simulink model "gru_FL"  (R2020a)
settings: Solver=FixedStepAuto  StartTime=0.0  StopTime=Inf  FixedStep=0.001  MaxStep=0.01  RelTol=1e-3
InitFcn:
  | init_gru
StopFcn:
  | %stop_gru
values from neighbouring files (symbols this model uses):
  centro = [points(1); points(2)]    [init_gru.m]
  K1 = [20; 20]    [init_gru.m]
  K2 = [100; 100]    [init_gru.m]
  K3 = [10; 10]    [init_gru.m]
  L_dot_iniziale = 0    [init_gru.m]
  L_iniziale = 2    [init_gru.m]
  Lsofar = [Lsofar; sum(Lenghts)]    [init_gru.m]
  Ltot = sum(Lenghts)    [init_gru.m]
  n_p = length(points)    [init_gru.m]
  phi_dot_iniziale = 360/180*pi    (= 6.28318530718)    [init_gru.m]
  phi_iniziale = 30/180*pi    (= 0.523598775598)    [init_gru.m]
  theta_dot_iniziale = pi/8    (= 0.392699081699)    [init_gru.m]
  theta_iniziale = 20/180*pi    (= 0.349065850399)    [init_gru.m]
  theta_rette = [theta_rette ; theta_rette(n_p-2)+pi]    [init_gru.m]
  v_r = v_rif    (= 1)    [init_gru.m]
  x_M_finale = points(1)    [init_gru.m]
  x_M_iniziale = x_M_iniziale + offset_iniziale    [init_gru.m]
  x_t_dot_iniziale = 0    [init_gru.m]
  x_t_iniziale = 0    [init_gru.m]
  xp = points(:,1)    [init_gru.m]
  y_M_finale = points(2)    [init_gru.m]
  y_M_iniziale = y_M_iniziale + offset_iniziale*2    [init_gru.m]
  y_t_dot_iniziale = 0    [init_gru.m]
  y_t_iniziale = 0    [init_gru.m]
  yp = points(:,2)    [init_gru.m]
undefined symbols (not defined in the file or in its folder): indexclot, Lsofarclot
libraries: simulink x1
settings Model: Creator=Andrea_Ferroni  LastModifiedBy=Francesco

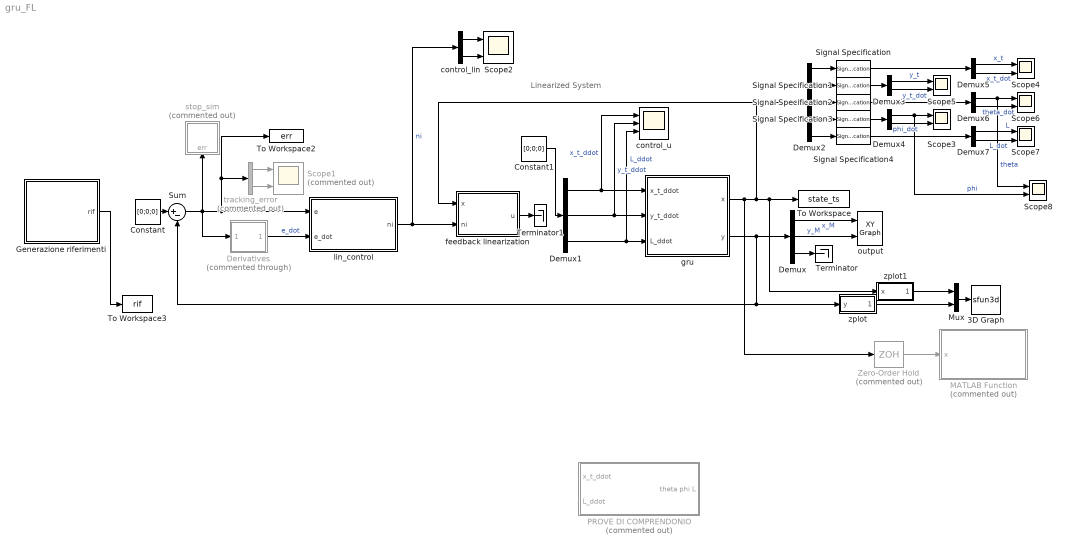
== system gru_FL ==
  note: Linearized System
  3D Graph : S-Function  LoadFcn=if exist('sfun3d','file'), sfun3d([],[],[],'LoadBlock'); end  FunctionName=sfun3d  Parameters=ax,T,np,cp,gd,ls,mk,mx,hd,tb  SFunctionDeploymentMode=off  EnableBusSupport=off  mask(3D Graph){np=2, ax=[-3 3 -3 3 -3 0.5], mx=1e4, T=0.1, cp=[3 2 1], gd=on, hd=off, tb=off, ls=-, mk=none}
      mask prompts: np "Number of moving points (lines)"; ax "Range: [xmin xmax  ymin ymax zmin zmax]"; mx "Max number of points in each line"; T "Sampling Time"; cp "Camera position (use [0 0 1] for 2D XY view)"; gd "Grid (on|off)"; hd "HeadMarkers (on|off)"; tb "Toolbar (on|off)"; ls "LineStyle"; mk "LineMarker"
      mask help:
      | This block plots the position of several points in the XYZ space. The input contains the coordinates of all the points (x1,y1,z1,x2,y2,z2,...).
      | The number of moving points (lines), the XYZ ranges, sampling time, camera position, and grid (among other things) can be set as mask parameters.
      settings: CopyFcn=if exist('sfun3d','file'), sfun3d([],[],[],'CopyBlock'); end  DeleteFcn=if exist('sfun3d','file'), sfun3d([],[],[],'DeleteBlock'); end  NameChangeFcn=if exist('sfun3d','file'), sfun3d([],[],[],'NameChange'); end
      mask Help:
      | This block plots the position of several points in the XYZ space. The input contains the coordinates of all the points (x1,y1,z1,x2,y2,z2,...).
      | The number of moving points (lines), the XYZ ranges, sampling time, camera position, and grid (among other things) can be set as mask parameters.
      mask TypeOptions ls: - | -- | : | -. | none
      mask TypeOptions mk: none | . | + | o | * | x | square | diamond | v | ^ | > | < | pentagram | hexagram
      mask Display: plot([.05 .95 .95 .05 .05],[.45 .45 .95 .95 .45], 0.5+cos(0:0.1:2*pi)*0.3,0.7+sin(0:0.1:2*pi)*0.2)
  Constant : Constant  Value=[0;0;0]
  Constant1 : Constant  Value=[0;0;0]
  Demux : Demux  Outputs=3
  Demux1 : Demux  Outputs=3
  Demux2 : Demux  Outputs=5
  Demux{3..7} (5 alike) : Demux  Outputs=2
  Derivatives : Subsystem  Commented=through
  Generazione riferimenti : Subsystem  Variant=on
  MATLAB Function : MATLAB Function  Commented=on  TreatAsAtomicUnit=on
  Mux : Mux  Inputs=2
  PROVE DI COMPRENDONIO : Subsystem  Commented=on
  Scope1 : Scope  Commented=on  NumInputPorts=2
  Scope{2..8} (7 alike) : Scope  NumInputPorts=2
  Signal Specification{,1..4} (5 alike) : SignalSpecification  Dimensions=[2,1]
  Sum : Sum  Inputs=|+-
  Terminator : Terminator
  Terminator1 : Terminator
  To Workspace : ToWorkspace  VariableName=state_ts  SaveFormat=Timeseries  SampleTime=-1
  To Workspace2 : ToWorkspace  VariableName=err  SaveFormat=Timeseries  SampleTime=-1
  To Workspace3 : ToWorkspace  VariableName=rif  SaveFormat=Timeseries  SampleTime=-1
  Zero-Order Hold : ZeroOrderHold  Commented=on  SampleTime=1/10
  control_lin : Demux  Outputs=2
  control_u : Scope  NumInputPorts=3
  feedback linearization : MATLAB Function  TreatAsAtomicUnit=on
  gru : Subsystem
  lin_control : MATLAB Function  TreatAsAtomicUnit=on
  output : simulink/Sinks/XY Graph  xmin=-50  xmax=50  ymin=-50  ymax=50  st=-1
  stop_sim : Subsystem  Commented=on
  tracking_error : Demux  Commented=on  Outputs=2
  zplot : MATLAB Function  TreatAsAtomicUnit=on
  zplot1 : MATLAB Function  TreatAsAtomicUnit=on
  wires:
  gru/2(y) -> Sum/2, zplot/1(y), Demux/1
  lin_control/1(ni) -> control_lin/1, feedback linearization/2(ni)  "ni"
  Sum/1 -> Derivatives/1(In1), lin_control/1(e), tracking_error/1, To Workspace2/1, stop_sim/1(err)
  Derivatives/1(Out1) -> lin_control/2(e_dot)  "e_dot"
  Demux/1 -> output/1  "x_M"
  Demux/2 -> output/2  "y_M"
  tracking_error/1 -> Scope1/1
  tracking_error/2 -> Scope1/2
  Demux1/1 -> control_u/1, gru/1(x_t_ddot)  "x_t_ddot"
  Demux1/2 -> gru/2(y_t_ddot), control_u/2  "y_t_ddot"
  control_lin/2 -> Scope2/2
  control_lin/1 -> Scope2/1
  Generazione riferimenti/1(rif) -> To Workspace3/1
  Demux1/3 -> control_u/3, gru/3(L_ddot)  "L_ddot"
  Demux/3 -> Terminator/1
  Demux2/1 -> Signal Specification/1
  Demux2/2 -> Signal Specification1/1
  Signal Specification1/1 -> Demux3/1
  Demux2/3 -> Signal Specification2/1
  Demux2/4 -> Signal Specification3/1
  Demux2/5 -> Signal Specification4/1
  Demux3/1 -> Scope5/1  "y_t"
  Demux3/2 -> Scope5/2  "y_t_dot"
  Demux4/1 -> Scope8/2, Scope3/1  "phi"
  Demux4/2 -> Scope3/2  "phi_dot"
  Signal Specification3/1 -> Demux4/1
  Demux5/1 -> Scope4/1  "x_t"
  Demux5/2 -> Scope4/2  "x_t_dot"
  Signal Specification/1 -> Demux5/1
  Demux6/1 -> Scope8/1, Scope6/1  "theta"
  Demux6/2 -> Scope6/2  "theta_dot"
  Signal Specification2/1 -> Demux6/1
  Demux7/1 -> Scope7/1  "L"
  Demux7/2 -> Scope7/2  "L_dot"
  Signal Specification4/1 -> Demux7/1
  Constant/1 -> Sum/1
  Constant1/1 -> Demux1/1
  zplot/1(y_new) -> Mux/2
  Mux/1 -> 3D Graph/1
  zplot1/1(trailer_graph) -> Mux/1
  gru/1(x) -> Zero-Order Hold/1, feedback linearization/1(x), Demux2/1, zplot1/1(x), To Workspace/1
  Zero-Order Hold/1 -> MATLAB Function/1(x)
  feedback linearization/1(u) -> Terminator1/1

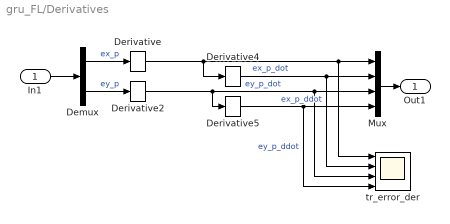
== system gru_FL/Derivatives ==
  In1 : Inport
  Demux : Demux  Outputs=2
  Derivative{,2,4..5} (4 alike) : Derivative  CoefficientInTFapproximation=1e10
  Mux : Mux
  tr_error_der : Scope  NumInputPorts=4
  Out1 : Outport
  wires:
  In1/1 -> Demux/1
  Demux/1 -> Derivative/1  "ex_p"
  Derivative/1 -> Derivative4/1, tr_error_der/1, Mux/1  "ex_p_dot"
  Demux/2 -> Derivative2/1  "ey_p"
  Mux/1 -> Out1/1
  Derivative4/1 -> tr_error_der/2, Mux/2  "ex_p_ddot"
  Derivative2/1 -> Derivative5/1, tr_error_der/3, Mux/3  "ey_p_dot"
  Derivative5/1 -> tr_error_der/4, Mux/4  "ey_p_ddot"

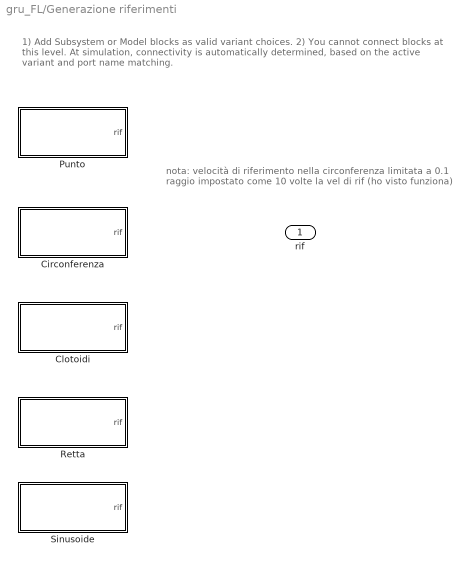
== system gru_FL/Generazione riferimenti ==
  note: nota:
      | velocità di riferimento nella circonferenza limitata a 0.1
      | raggio impostato come 10 volte la vel di rif (ho visto funziona)
  note: 1) Add Subsystem or Model blocks as valid variant choices.
      | 2) You cannot connect blocks at this level. At simulation, connectivity is automatically
      | determined, based on the active variant and port name matching.
  Circonferenza : Subsystem  VariantControl=Circonferenza
  Clotoidi : Subsystem  VariantControl=Clotoidi
  Punto : Subsystem  VariantControl=Punto
  Retta : Subsystem  VariantControl=Retta
  Sinusoide : Subsystem  VariantControl=Sinusoide
  rif : Outport

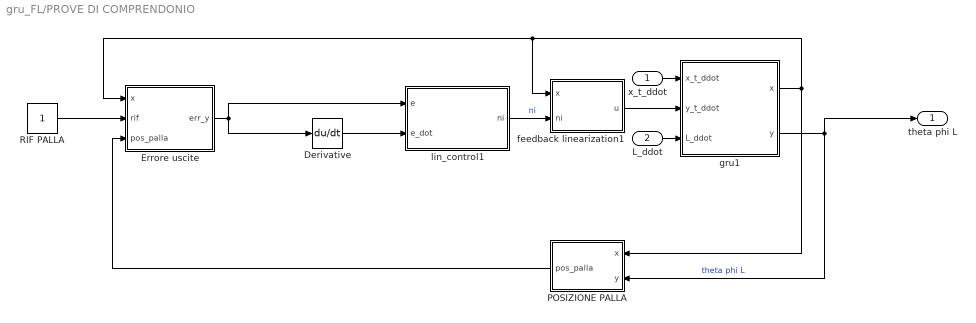
== system gru_FL/PROVE DI COMPRENDONIO ==
  x_t_ddot : Inport
  L_ddot : Inport  Port=2
  Derivative : Derivative
  Errore uscite : MATLAB Function  TreatAsAtomicUnit=on
  POSIZIONE PALLA : MATLAB Function  TreatAsAtomicUnit=on
  RIF PALLA : Constant
  feedback linearization1 : MATLAB Function  TreatAsAtomicUnit=on
  gru1 : Subsystem
  lin_control1 : MATLAB Function  TreatAsAtomicUnit=on
  theta phi L : Outport
  wires:
  Derivative/1 -> lin_control1/2(e_dot)
  lin_control1/1(ni) -> feedback linearization1/2(ni)  "ni"
  gru1/2(y) -> theta phi L/1, POSIZIONE PALLA/2(y)  "theta phi L"
  x_t_ddot/1 -> gru1/1(x_t_ddot)
  Errore uscite/1(err_y) -> lin_control1/1(e), Derivative/1
  POSIZIONE PALLA/1(pos_palla) -> Errore uscite/3(pos_palla)
  RIF PALLA/1 -> Errore uscite/2(rif)
  gru1/1(x) -> POSIZIONE PALLA/1(x), Errore uscite/1(x), feedback linearization1/1(x)
  feedback linearization1/1(u) -> gru1/2(y_t_ddot)
  L_ddot/1 -> gru1/3(L_ddot)

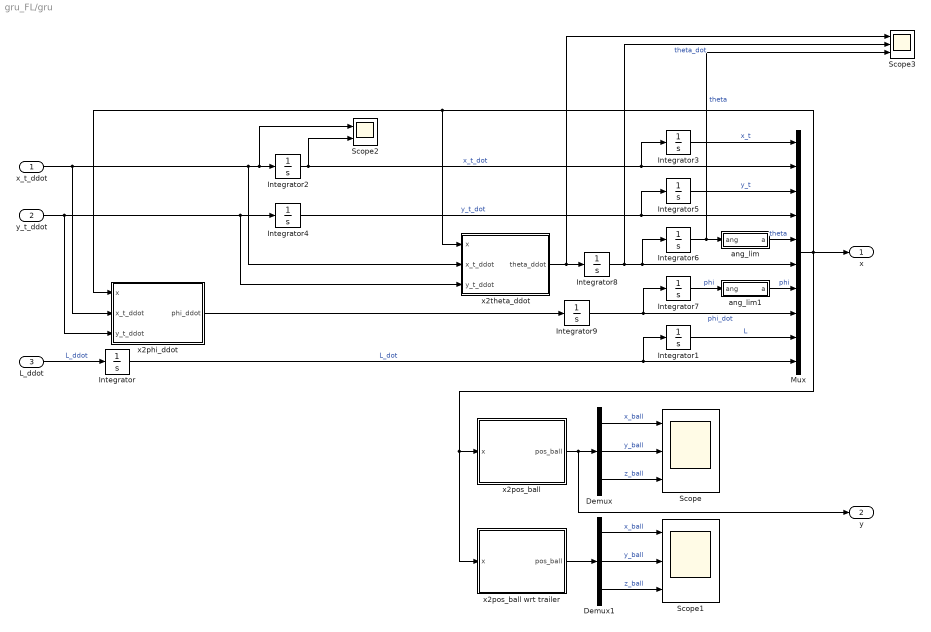
== system gru_FL/gru ==
  x_t_ddot : Inport
  y_t_ddot : Inport  Port=2
  L_ddot : Inport  Port=3
  Demux : Demux  Outputs=3
  Demux1 : Demux  Outputs=3
  Integrator : Integrator  InitialCondition=L_dot_iniziale
  Integrator1 : Integrator  InitialCondition=L_iniziale
  Integrator2 : Integrator  InitialCondition=x_t_dot_iniziale  UpperSaturationLimit=1e3  LowerSaturationLimit=-1e3
  Integrator3 : Integrator  InitialCondition=x_t_iniziale
  Integrator4 : Integrator  InitialCondition=y_t_dot_iniziale
  Integrator5 : Integrator  InitialCondition=y_t_iniziale
  Integrator6 : Integrator  InitialCondition=theta_iniziale
  Integrator7 : Integrator  InitialCondition=phi_iniziale
  Integrator8 : Integrator  InitialCondition=theta_dot_iniziale
  Integrator9 : Integrator  InitialCondition=phi_dot_iniziale
  Mux : Mux  Inputs=10
  Scope : Scope  NumInputPorts=3
  Scope1 : Scope  NumInputPorts=3
  Scope2 : Scope  NumInputPorts=2
  Scope3 : Scope  NumInputPorts=3
  ang_lim : MATLAB Function  TreatAsAtomicUnit=on
  ang_lim1 : MATLAB Function  TreatAsAtomicUnit=on
  x2phi_ddot : MATLAB Function  TreatAsAtomicUnit=on
  x2pos_ball : MATLAB Function  TreatAsAtomicUnit=on
  x2pos_ball wrt trailer : MATLAB Function  TreatAsAtomicUnit=on
  x2theta_ddot : MATLAB Function  TreatAsAtomicUnit=on
  x : Outport
  y : Outport  Port=2
  wires:
  x2pos_ball/1(pos_ball) -> y/1, Demux/1
  Integrator3/1 -> Mux/1  "x_t"
  Integrator2/1 -> Scope2/2, Integrator3/1, Mux/2  "x_t_dot"
  Integrator5/1 -> Mux/3  "y_t"
  Integrator4/1 -> Integrator5/1, Mux/4  "y_t_dot"
  Integrator6/1 -> Scope3/3, ang_lim/1(ang)  "theta"
  Integrator8/1 -> Scope3/2, Integrator6/1, Mux/6  "theta_dot"
  Integrator7/1 -> ang_lim1/1(ang)  "phi"
  Integrator9/1 -> Integrator7/1, Mux/8  "phi_dot"
  Integrator1/1 -> Mux/9  "L"
  L_ddot/1 -> Integrator/1  "L_ddot"
  Demux/1 -> Scope/1  "x_ball"
  Demux/2 -> Scope/2  "y_ball"
  Demux/3 -> Scope/3  "z_ball"
  Integrator/1 -> Integrator1/1, Mux/10  "L_dot"
  x_t_ddot/1 -> x2theta_ddot/2(x_t_ddot), Scope2/1, Integrator2/1, x2phi_ddot/2(x_t_ddot)
  y_t_ddot/1 -> x2theta_ddot/3(y_t_ddot), Integrator4/1, x2phi_ddot/3(y_t_ddot)
  x2theta_ddot/1(theta_ddot) -> Scope3/1, Integrator8/1
  x2phi_ddot/1(phi_ddot) -> Integrator9/1
  Mux/1 -> x2pos_ball wrt trailer/1(x), x2pos_ball/1(x), x2phi_ddot/1(x), x2theta_ddot/1(x), x/1
  Demux1/3 -> Scope1/3  "z_ball"
  Demux1/2 -> Scope1/2  "y_ball"
  Demux1/1 -> Scope1/1  "x_ball"
  x2pos_ball wrt trailer/1(pos_ball) -> Demux1/1
  ang_lim/1(a) -> Mux/5  "theta"
  ang_lim1/1(a) -> Mux/7  "phi"

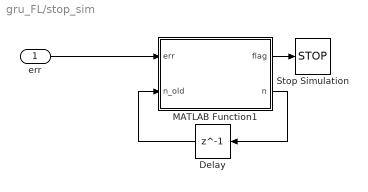
== system gru_FL/stop_sim ==
  err : Inport
  Delay : Delay  DelayLength=1
  MATLAB Function1 : MATLAB Function  TreatAsAtomicUnit=on
  Stop Simulation : Stop
  wires:
  MATLAB Function1/2(n) -> Delay/1
  MATLAB Function1/1(flag) -> Stop Simulation/1
  err/1 -> MATLAB Function1/1(err)
  Delay/1 -> MATLAB Function1/2(n_old)

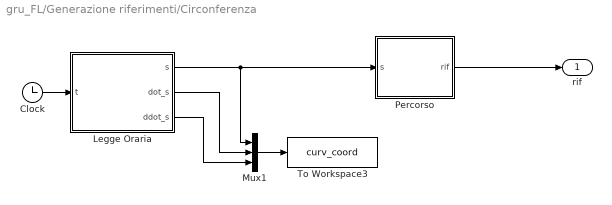
== system gru_FL/Generazione riferimenti/Circonferenza ==
  Clock : Clock
  Legge Oraria : MATLAB Function  TreatAsAtomicUnit=on
  Mux1 : Mux  Inputs=3
  Percorso : MATLAB Function  TreatAsAtomicUnit=on
  To Workspace3 : ToWorkspace  VariableName=curv_coord  SaveFormat=Timeseries  SampleTime=-1
  rif : Outport
  wires:
  Legge Oraria/2(dot_s) -> Mux1/2
  Clock/1 -> Legge Oraria/1(t)
  Mux1/1 -> To Workspace3/1
  Legge Oraria/3(ddot_s) -> Mux1/3
  Legge Oraria/1(s) -> Percorso/1(s), Mux1/1
  Percorso/1(rif) -> rif/1

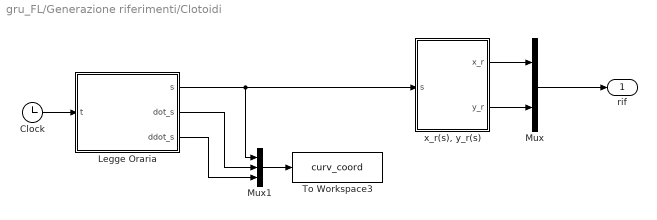
== system gru_FL/Generazione riferimenti/Clotoidi ==
  Clock : Clock
  Legge Oraria : MATLAB Function  TreatAsAtomicUnit=on
  Mux : Mux  Inputs=2
  Mux1 : Mux  Inputs=3
  To Workspace3 : ToWorkspace  VariableName=curv_coord  SaveFormat=Timeseries  SampleTime=-1
  "x_r(s), y_r(s)" : MATLAB Function  TreatAsAtomicUnit=on
  rif : Outport
  wires:
  Legge Oraria/1(s) -> Mux1/1, "x_r(s), y_r(s)"/1(s)
  Legge Oraria/2(dot_s) -> Mux1/2
  Clock/1 -> Legge Oraria/1(t)
  Legge Oraria/3(ddot_s) -> Mux1/3
  Mux1/1 -> To Workspace3/1
  "x_r(s), y_r(s)"/2(y_r) -> Mux/2
  "x_r(s), y_r(s)"/1(x_r) -> Mux/1
  Mux/1 -> rif/1

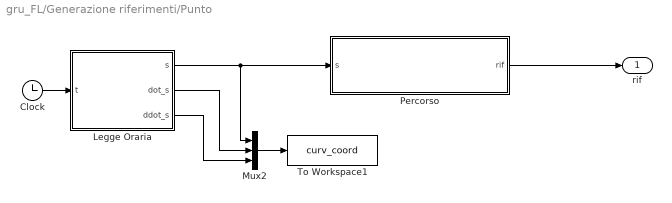
== system gru_FL/Generazione riferimenti/Punto ==
  Clock : Clock
  Legge Oraria : MATLAB Function  TreatAsAtomicUnit=on
  Mux2 : Mux  Inputs=3
  Percorso : MATLAB Function  TreatAsAtomicUnit=on
  To Workspace1 : ToWorkspace  VariableName=curv_coord  SaveFormat=Timeseries  SampleTime=-1
  rif : Outport
  wires:
  Legge Oraria/2(dot_s) -> Mux2/2
  Clock/1 -> Legge Oraria/1(t)
  Mux2/1 -> To Workspace1/1
  Legge Oraria/3(ddot_s) -> Mux2/3
  Legge Oraria/1(s) -> Mux2/1, Percorso/1(s)
  Percorso/1(rif) -> rif/1

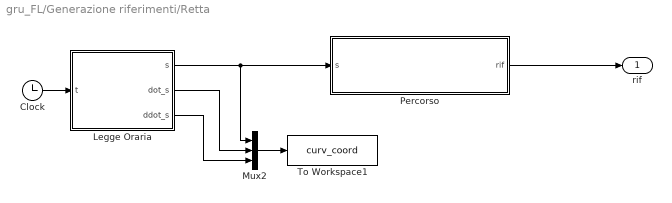
== system gru_FL/Generazione riferimenti/Retta ==
  Clock : Clock
  Legge Oraria : MATLAB Function  TreatAsAtomicUnit=on
  Mux2 : Mux  Inputs=3
  Percorso : MATLAB Function  TreatAsAtomicUnit=on
  To Workspace1 : ToWorkspace  VariableName=curv_coord  SaveFormat=Timeseries  SampleTime=-1
  rif : Outport
  wires:
  Percorso/1(rif) -> rif/1
  Legge Oraria/1(s) -> Percorso/1(s), Mux2/1
  Legge Oraria/3(ddot_s) -> Mux2/3
  Mux2/1 -> To Workspace1/1
  Clock/1 -> Legge Oraria/1(t)
  Legge Oraria/2(dot_s) -> Mux2/2

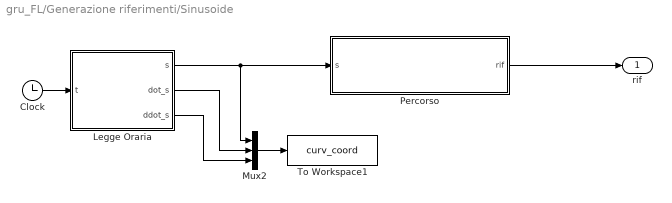
== system gru_FL/Generazione riferimenti/Sinusoide ==
  Clock : Clock
  Legge Oraria : MATLAB Function  TreatAsAtomicUnit=on
  Mux2 : Mux  Inputs=3
  Percorso : MATLAB Function  TreatAsAtomicUnit=on
  To Workspace1 : ToWorkspace  VariableName=curv_coord  SaveFormat=Timeseries  SampleTime=-1
  rif : Outport
  wires:
  Legge Oraria/2(dot_s) -> Mux2/2
  Clock/1 -> Legge Oraria/1(t)
  Mux2/1 -> To Workspace1/1
  Legge Oraria/3(ddot_s) -> Mux2/3
  Legge Oraria/1(s) -> Mux2/1, Percorso/1(s)
  Percorso/1(rif) -> rif/1

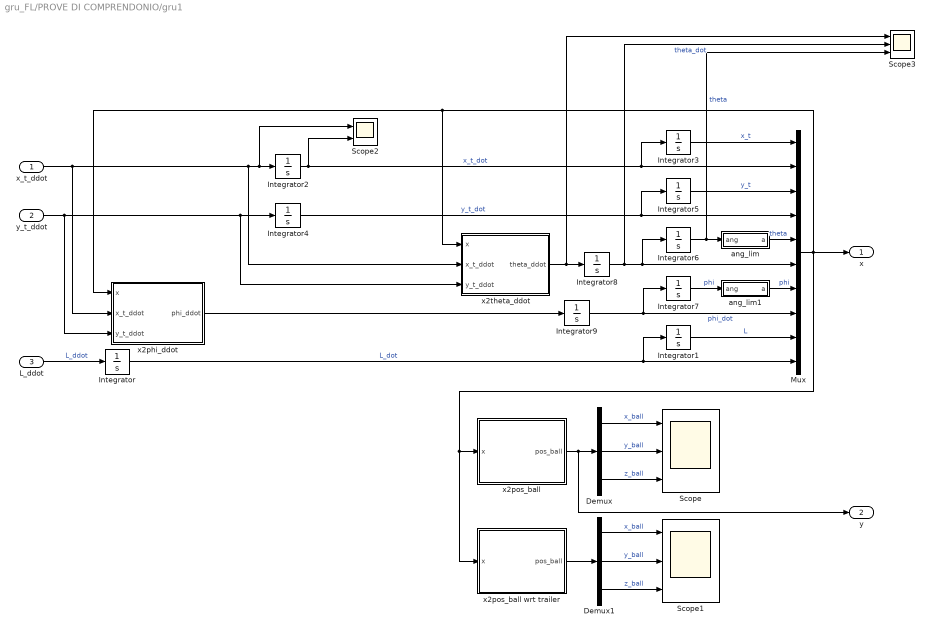
== system gru_FL/PROVE DI COMPRENDONIO/gru1 ==
  x_t_ddot : Inport
  y_t_ddot : Inport  Port=2
  L_ddot : Inport  Port=3
  Demux : Demux  Outputs=3
  Demux1 : Demux  Outputs=3
  Integrator : Integrator  InitialCondition=L_dot_iniziale
  Integrator1 : Integrator  InitialCondition=L_iniziale
  Integrator2 : Integrator  InitialCondition=x_t_dot_iniziale  UpperSaturationLimit=1e3  LowerSaturationLimit=-1e3
  Integrator3 : Integrator  InitialCondition=x_t_iniziale
  Integrator4 : Integrator  InitialCondition=y_t_dot_iniziale
  Integrator5 : Integrator  InitialCondition=y_t_iniziale
  Integrator6 : Integrator  InitialCondition=theta_iniziale
  Integrator7 : Integrator  InitialCondition=phi_iniziale
  Integrator8 : Integrator  InitialCondition=theta_dot_iniziale
  Integrator9 : Integrator  InitialCondition=phi_dot_iniziale
  Mux : Mux  Inputs=10
  Scope : Scope  NumInputPorts=3
  Scope1 : Scope  NumInputPorts=3
  Scope2 : Scope  NumInputPorts=2
  Scope3 : Scope  NumInputPorts=3
  ang_lim : MATLAB Function  TreatAsAtomicUnit=on
  ang_lim1 : MATLAB Function  TreatAsAtomicUnit=on
  x2phi_ddot : MATLAB Function  TreatAsAtomicUnit=on
  x2pos_ball : MATLAB Function  TreatAsAtomicUnit=on
  x2pos_ball wrt trailer : MATLAB Function  TreatAsAtomicUnit=on
  x2theta_ddot : MATLAB Function  TreatAsAtomicUnit=on
  x : Outport
  y : Outport  Port=2
  wires:
  ang_lim1/1(a) -> Mux/7  "phi"
  ang_lim/1(a) -> Mux/5  "theta"
  x2pos_ball wrt trailer/1(pos_ball) -> Demux1/1
  Demux1/1 -> Scope1/1  "x_ball"
  Demux1/2 -> Scope1/2  "y_ball"
  Demux1/3 -> Scope1/3  "z_ball"
  Mux/1 -> x/1, x2theta_ddot/1(x), x2phi_ddot/1(x), x2pos_ball/1(x), x2pos_ball wrt trailer/1(x)
  x2phi_ddot/1(phi_ddot) -> Integrator9/1
  x2theta_ddot/1(theta_ddot) -> Integrator8/1, Scope3/1
  y_t_ddot/1 -> x2phi_ddot/3(y_t_ddot), Integrator4/1, x2theta_ddot/3(y_t_ddot)
  x_t_ddot/1 -> x2phi_ddot/2(x_t_ddot), Integrator2/1, Scope2/1, x2theta_ddot/2(x_t_ddot)
  Integrator/1 -> Mux/10, Integrator1/1  "L_dot"
  Demux/3 -> Scope/3  "z_ball"
  Demux/2 -> Scope/2  "y_ball"
  Demux/1 -> Scope/1  "x_ball"
  L_ddot/1 -> Integrator/1  "L_ddot"
  Integrator1/1 -> Mux/9  "L"
  Integrator9/1 -> Mux/8, Integrator7/1  "phi_dot"
  Integrator7/1 -> ang_lim1/1(ang)  "phi"
  Integrator8/1 -> Mux/6, Integrator6/1, Scope3/2  "theta_dot"
  Integrator6/1 -> ang_lim/1(ang), Scope3/3  "theta"
  Integrator4/1 -> Mux/4, Integrator5/1  "y_t_dot"
  Integrator5/1 -> Mux/3  "y_t"
  Integrator2/1 -> Mux/2, Integrator3/1, Scope2/2  "x_t_dot"
  Integrator3/1 -> Mux/1  "x_t"
  x2pos_ball/1(pos_ball) -> Demux/1, y/1

== matlab function gru_FL/Generazione riferimenti/Clotoidi/Legge Oraria ==
  data: t input; s output; v_rif parameter; dot_s output; ddot_s output
function [s, dot_s, ddot_s]  = legge_oraria(t, v_rif)
%#codegen PEPO

s = v_rif*t;
dot_s = v_rif;
ddot_s = 0.0;


end

== matlab function gru_FL/gru/x2phi_ddot ==
  data: x input; phi_ddot output; x_t_ddot input; y_t_ddot input
function phi_ddot = fcn(x, x_t_ddot, y_t_ddot)
	
	theta		= x(5);
	theta_dot	= x(6);
	phi			= x(7);
	phi_dot		= x(8);
	L			= x(9);
	L_dot		= x(10);
	
phi_ddot = -2*(L_dot/L)*phi_dot-2*phi_dot*theta_dot*cot(theta) + (-cos(phi)/(sin(theta)*L))*x_t_ddot + (sin(phi)/(sin(theta)*L))*y_t_ddot;

== matlab function gru_FL/Generazione riferimenti/Circonferenza/Legge Oraria ==
  data: t input; s output; v_rif parameter; dot_s output; ddot_s output
function [s, dot_s, ddot_s]  = legge_oraria(t, v_rif)
%#codegen PEPO

s = v_rif*t;
dot_s = v_rif;
ddot_s = 0.0;


end

== matlab function gru_FL/Generazione riferimenti/Circonferenza/Percorso ==
  data: s input; rif output; centro parameter; v_r parameter
function rif = percorso(s, centro, v_r)

r = 10*v_r;  % 1
theta_circ = s/r;

if theta_circ >=  3*2*pi % dopotre giri ti fermi
	theta_circ = 3*2*pi;
end

rif = centro + r*[cos(theta_circ);sin(theta_circ)];		% circonferenza

end

== matlab function gru_FL/Generazione riferimenti/Retta/Legge Oraria ==
  data: t input; s output; v_rif parameter; dot_s output; ddot_s output
function [s, dot_s, ddot_s]  = legge_oraria(t, v_rif)
%#codegen PEPO

s = v_rif*t;
dot_s = v_rif;
ddot_s = 0.0;


end

== matlab function gru_FL/Generazione riferimenti/Retta/Percorso ==
  data: s input; rif output; dir_retta parameter
function rif  = retta(s, dir_retta)

rif = [0;0] + s * dir_retta;


end

== matlab function gru_FL/Generazione riferimenti/Clotoidi/x_r(s), y_r(s) ==
  data: s input; x_r output size=1; y_r output size=1; indexclot parameter; theta_rette parameter; yp parameter; xp parameter; Lsofar parameter; n_p parameter; Lsofarclot parameter; Ltot parameter
function [x_r,y_r] = percorso(s, indexclot, theta_rette, yp, xp, ...
										Lsofar, n_p, Lsofarclot, Ltot)
									
coder.extrinsic('pointsOnClothoid')
% fine percorso
if s >= Ltot
	s = Ltot; % cosi` da plottare l'ultimo punto
end

ntratto=0;
	XYS = [0; 0]; %definito prima

	%Parte per capire in che tratto sono
	if s < Lsofar(1)
		ntratto=1;
	else
		for ii=2:(n_p-1)
			if s>=Lsofar(ii-1) && s<=Lsofar(ii)
				ntratto=ii;
			end
		end
	end	

		%calcolo delle coordinate x e y riferite a s e a ntratto
	if mod(ntratto,2)==1            %tratti dispari - rette
		if ntratto==1
			XYS=[xp(ntratto)+cos(theta_rette(ntratto))*(s); ...
				yp(ntratto)+sin(theta_rette(ntratto))*(s)];
		else
			srel=s-Lsofar(ntratto-1);
			XYS=[	xp(ntratto)	+ cos(theta_rette(ntratto))	* srel; ...
					yp(ntratto)	+ sin(theta_rette(ntratto))	* srel];
		end 

	elseif mod(ntratto,2)==0	%tratti pari - clotoidi
		srel=s-Lsofar(ntratto-1);

		if srel<=Lsofarclot(ntratto/2).Lclot(1)
			XYS = double(pointsOnClothoid( indexclot(ntratto/2).clot.S0, srel ));

		elseif srel>Lsofarclot(ntratto/2).Lclot(1) & srel<=Lsofarclot(ntratto/2).Lclot(2)
			XYS = double(pointsOnClothoid( indexclot(ntratto/2).clot.SM, srel- indexclot(ntratto/2).clot.S0.L ));

		elseif srel>Lsofarclot(ntratto/2).Lclot(2)
			XYS = double(pointsOnClothoid( indexclot(ntratto/2).clot.S1, srel- indexclot(ntratto/2).clot.S0.L - indexclot(ntratto/2).clot.SM.L ));
		end

		%XYS = double(pointsOnClothoid( indexclot(ntratto/2).clot, s-Lsofar(ntratto-1) ));
	end

	x_r = XYS(1);
	y_r = XYS(2);
%--------------------------------------------------
% end function
end

== matlab function gru_FL/Generazione riferimenti/Sinusoide/Legge Oraria ==
  data: t input; s output; v_rif parameter; dot_s output; ddot_s output
function [s, dot_s, ddot_s]  = legge_oraria(t, v_rif)
%#codegen PEPO

s = v_rif*t;
dot_s = v_rif;
ddot_s = 0.0;


end

== matlab function gru_FL/Generazione riferimenti/Sinusoide/Percorso ==
  data: s input; rif output; dir_retta parameter
function rif  = retta(s, dir_retta)

r = 5;
theta_circ = s/r;

% if theta_circ >=  3*2*pi % dopotre giri ti fermi
% 	theta_circ = 3*2*pi;
% end

rif = dir_retta * s + r*[0; sin(theta_circ)];	% circonferenza

end

== matlab function gru_FL/gru/x2pos_ball ==
  data: x input; pos_ball output; z_t parameter
function pos_ball = fcn(x, z_t)
	
	x_t		= x(1);
	y_t		= x(3);
	theta	= x(5);
	phi		= x(7);
	L		= x(9);
	
pos_ball = [x_t + L*sin(theta)*sin(phi); ...
			y_t + L*sin(theta)*cos(phi);...
			z_t + L*cos(theta)];

== matlab function gru_FL/gru/x2pos_ball wrt trailer ==
  data: x input; pos_ball output
function pos_ball = fcn(x)
	
	theta	= x(5);
	phi		= x(7);
	L		= x(9);
	
pos_ball = [ L*sin(theta)*sin(phi); ...
			 L*sin(theta)*cos(phi);...
			 L*cos(theta)];

== matlab function gru_FL/gru/ang_lim ==
  data: ang input; a output
function a = ang_lim(ang)

	c = cos(ang);
	s = sin(ang);
	a = atan2(s, c);

end

== matlab function gru_FL/gru/ang_lim1 ==
  data: ang input; a output
function a = ang_lim(ang)

	c = cos(ang);
	s = sin(ang);
	a = atan2(s, c);

end

== matlab function gru_FL/zplot ==
  data: y input; y_new output
function y_new = fcn(y)

y_new	 = y;
y_new(3) = -y_new(3);

end

== matlab function gru_FL/zplot1 ==
  data: x input; trailer_graph output; z_t parameter
function trailer_graph = fcn(x, z_t)

	trailer_graph = [x(1); x(3); z_t];

end

== matlab function gru_FL/MATLAB Function ==
  data: x input; z_t parameter
function gru_plot(x, z_t)

coder.extrinsic('plot3')
coder.extrinsic('text')
coder.extrinsic('num2str')

% get relevant signals
x_t		= x(1);
y_t		= x(3);
theta	= x(5);
phi		= x(7);
L		= x(9);

% get mass position
pos_ball = [ L*sin(theta)*sin(phi); ...
			 L*sin(theta)*cos(phi);...
			 -L*cos(theta)];

% figure
figure(1)
plot3(x_t, y_t, -z_t, 'bd', 'MarkerSize', 5)
hold on
plot3(pos_ball(1), pos_ball(2), pos_ball(3), 'ro', 'MarkerSize', 5)
plot3([x_t, pos_ball(1)], [y_t, pos_ball(2)], [-z_t, pos_ball(3)], 'k-', 'LineWidth', 2)
text(0,0,0,['theta ' num2str(theta/pi*180)])
grid on
view([45 10])
xlim([-3 3])
xlabel('X')
ylim([-3 3])
ylabel('Y')
zlim([-3 0.5])
zlabel('Z')
hold off
drawnow

end

== matlab function gru_FL/PROVE DI COMPRENDONIO/gru1/ang_lim ==
  data: ang input; a output
function a = ang_lim(ang)

	c = cos(ang);
	s = sin(ang);
	a = atan2(s, c);

end

== matlab function gru_FL/PROVE DI COMPRENDONIO/gru1/ang_lim1 ==
  data: ang input; a output
function a = ang_lim(ang)

	c = cos(ang);
	s = sin(ang);
	a = atan2(s, c);

end

== matlab function gru_FL/PROVE DI COMPRENDONIO/gru1/x2phi_ddot ==
  data: x input; phi_ddot output; x_t_ddot input; y_t_ddot input
function phi_ddot = fcn(x, x_t_ddot, y_t_ddot)
	
	theta		= x(5);
	theta_dot	= x(6);
	phi			= x(7);
	phi_dot		= x(8);
	L			= x(9);
	L_dot		= x(10);
	
phi_ddot = -2*(L_dot/L)*phi_dot-2*phi_dot*theta_dot*cot(theta) + (-cos(phi)/(sin(theta)*L))*x_t_ddot + (sin(phi)/(sin(theta)*L))*y_t_ddot;

== matlab function gru_FL/PROVE DI COMPRENDONIO/gru1/x2pos_ball ==
  data: x input; pos_ball output; z_t parameter
function pos_ball = fcn(x, z_t)
	
	x_t		= x(1);
	y_t		= x(3);
	theta	= x(5);
	phi		= x(7);
	L		= x(9);
	
pos_ball = [x_t + L*sin(theta)*sin(phi); ...
			y_t + L*sin(theta)*cos(phi);...
			z_t + L*cos(theta)];

== matlab function gru_FL/PROVE DI COMPRENDONIO/gru1/x2pos_ball wrt trailer ==
  data: x input; pos_ball output
function pos_ball = fcn(x)
	
	theta	= x(5);
	phi		= x(7);
	L		= x(9);
	
pos_ball = [ L*sin(theta)*sin(phi); ...
			 L*sin(theta)*cos(phi);...
			 L*cos(theta)];

== matlab function gru_FL/PROVE DI COMPRENDONIO/gru1/x2theta_ddot ==
  data: x input; theta_ddot output; x_t_ddot input; y_t_ddot input; g parameter
function theta_ddot = fcn(x, x_t_ddot, y_t_ddot, g)
	
	theta		= x(5);
	theta_dot	= x(6);
	phi			= x(7);
	phi_dot		= x(8);
	L			= x(9);
	L_dot		= x(10);
	
theta_ddot = -2*(L_dot/L)*theta_dot+0.5*phi_dot^2*sin(2*theta)-(g/L)*sin(theta) + (-cos(theta)*sin(phi)/L)*x_t_ddot + (-cos(theta)*cos(phi)/L)*y_t_ddot;

== matlab function gru_FL/PROVE DI COMPRENDONIO/feedback linearization1 ==
  data: x input; ni input; u output
function u = Linearized(x,ni)
E_inv = inv_E(x);
G = Gamma(x);
u =  -E_inv*G + E_inv*ni;
end

% gamma
function Gm = Gamma(x)
	theta		= x(5);
	theta_dot	= x(6);
	phi			= x(7);
	phi_dot		= x(8);
	L			= x(9);

% Gm_tot =  L_dot*(phi_dot*cos(phi)*sin(theta) + theta_dot*cos(theta)*sin(phi)) + phi_dot*(L_dot*cos(phi)*sin(theta) + L*theta_dot*cos(phi)*cos(theta) - L*phi_dot*sin(phi)*sin(theta)) + theta_dot*(L_dot*cos(theta)*sin(phi) + L*phi_dot*cos(phi)*cos(theta) - L*theta_dot*sin(phi)*sin(theta)) - L*cos(phi)*sin(theta)*(2*phi_dot*theta_dot*cot(theta) + (2*L_dot*phi_dot)/L) - L*cos(theta)*sin(phi)*((981*sin(theta))/(100*L) - (phi_dot^2*sin(2*theta))/2 + (2*L_dot*theta_dot)/L)
%  L_dot*(theta_dot*cos(phi)*cos(theta) - phi_dot*sin(phi)*sin(theta)) - theta_dot*(L*phi_dot*cos(theta)*sin(phi) - L_dot*cos(phi)*cos(theta) + L*theta_dot*cos(phi)*sin(theta)) - phi_dot*(L_dot*sin(phi)*sin(theta) + L*phi_dot*cos(phi)*sin(theta) + L*theta_dot*cos(theta)*sin(phi)) + L*sin(phi)*sin(theta)*(2*phi_dot*theta_dot*cot(theta) + (2*L_dot*phi_dot)/L) - L*cos(phi)*cos(theta)*((981*sin(theta))/(100*L) - (phi_dot^2*sin(2*theta))/2 + (2*L_dot*theta_dot)/L)
%                                                                                                                                                                                                                                                                                             L*sin(theta)*((981*sin(theta))/(100*L) - (phi_dot^2*sin(2*theta))/2 + (2*L_dot*theta_dot)/L) - L_dot*theta_dot*sin(theta) - theta_dot*(L_dot*sin(theta) + L*theta_dot*cos(theta))

Gm =[-(sin(phi)*sin(theta)*(981*cos(theta) + 100*L*phi_dot^2 + 100*L*theta_dot^2 - 100*L*phi_dot^2*cos(theta)^2))/100;...
	 -(cos(phi)*sin(theta)*(981*cos(theta) + 100*L*phi_dot^2 + 100*L*theta_dot^2 - 100*L*phi_dot^2*cos(theta)^2))/100;...
	 L*phi_dot^2*cos(theta)^3 - L*phi_dot^2*cos(theta) - L*theta_dot^2*cos(theta) - (981*cos(theta)^2)/100 + 981/100];
 
end
% 
function E_in = inv_E(x)
	theta		= x(5);
	phi			= x(7);
	L			= x(9); 
	
E =[1 - cos(theta)^2*sin(phi)^2 - cos(phi)^2,			cos(phi)*sin(phi) - cos(phi)*cos(theta)^2*sin(phi),	sin(phi)*sin(theta);...
	cos(phi)*sin(phi) - cos(phi)*cos(theta)^2*sin(phi),	1 - cos(phi)^2*cos(theta)^2 - sin(phi)^2,			cos(phi)*sin(theta);...
	cos(theta)*sin(phi)*sin(theta),						cos(phi)*cos(theta)*sin(theta),						cos(theta)];

E_in = inv(E);



E_BIS = [	1 - cos(theta)^2*sin(phi)^2 - cos(phi)^2,			  cos(phi)*sin(phi) - cos(phi)*cos(theta)^2*sin(phi),    sin(phi)*sin(theta);...
			cos(phi)*sin(phi) - cos(phi)*cos(theta)^2*sin(phi),				1 - cos(phi)^2*cos(theta)^2 - sin(phi)^2,    cos(phi)*sin(theta);...
            -(cos(theta)*sin(phi))/L,														-(cos(phi)*cos(theta))/L,                     0];


if rcond(E_BIS) < 1e-3
	ciao = 1;
	%rcond(E_BIS)
	%rcond(E)
end

end

== matlab function gru_FL/PROVE DI COMPRENDONIO/lin_control1 ==
  data: e input; ni output; e_dot input; K1 parameter; K2 parameter; K3 parameter
function ni = lin_control(e, e_dot, K1, K2, K3)


% ni = K1.*e + K2.*edot + K3.*eddot;
ni = [0; 0; 0];

end

== matlab function gru_FL/PROVE DI COMPRENDONIO/POSIZIONE PALLA ==
  data: x input; pos_palla output; y input
function pos_palla = fcn(x, y)

y = u;

== matlab function gru_FL/PROVE DI COMPRENDONIO/Errore uscite ==
  data: x input; rif input; err_y output; pos_palla input
function err_y = fcn(x, rif, pos_palla)

y = u;

== matlab function gru_FL/lin_control ==
  data: e input; ni output; e_dot input; K1 parameter; K2 parameter; K3 parameter
function ni = lin_control(e, e_dot, K1, K2, K3)


% ni = K1.*e + K2.*edot + K3.*eddot;
ni = [0; 0; 0];

end

== matlab function gru_FL/feedback linearization ==
  data: x input; ni input; u output
function u = Linearized(x,ni)
E_inv = inv_E(x);
G = Gamma(x);
u =  -E_inv*G + E_inv*ni;
end

% gamma
function Gm = Gamma(x)
	theta		= x(5);
	theta_dot	= x(6);
	phi			= x(7);
	phi_dot		= x(8);
	L			= x(9);

% Gm_tot =  L_dot*(phi_dot*cos(phi)*sin(theta) + theta_dot*cos(theta)*sin(phi)) + phi_dot*(L_dot*cos(phi)*sin(theta) + L*theta_dot*cos(phi)*cos(theta) - L*phi_dot*sin(phi)*sin(theta)) + theta_dot*(L_dot*cos(theta)*sin(phi) + L*phi_dot*cos(phi)*cos(theta) - L*theta_dot*sin(phi)*sin(theta)) - L*cos(phi)*sin(theta)*(2*phi_dot*theta_dot*cot(theta) + (2*L_dot*phi_dot)/L) - L*cos(theta)*sin(phi)*((981*sin(theta))/(100*L) - (phi_dot^2*sin(2*theta))/2 + (2*L_dot*theta_dot)/L)
%  L_dot*(theta_dot*cos(phi)*cos(theta) - phi_dot*sin(phi)*sin(theta)) - theta_dot*(L*phi_dot*cos(theta)*sin(phi) - L_dot*cos(phi)*cos(theta) + L*theta_dot*cos(phi)*sin(theta)) - phi_dot*(L_dot*sin(phi)*sin(theta) + L*phi_dot*cos(phi)*sin(theta) + L*theta_dot*cos(theta)*sin(phi)) + L*sin(phi)*sin(theta)*(2*phi_dot*theta_dot*cot(theta) + (2*L_dot*phi_dot)/L) - L*cos(phi)*cos(theta)*((981*sin(theta))/(100*L) - (phi_dot^2*sin(2*theta))/2 + (2*L_dot*theta_dot)/L)
%                                                                                                                                                                                                                                                                                             L*sin(theta)*((981*sin(theta))/(100*L) - (phi_dot^2*sin(2*theta))/2 + (2*L_dot*theta_dot)/L) - L_dot*theta_dot*sin(theta) - theta_dot*(L_dot*sin(theta) + L*theta_dot*cos(theta))

Gm =[-(sin(phi)*sin(theta)*(981*cos(theta) + 100*L*phi_dot^2 + 100*L*theta_dot^2 - 100*L*phi_dot^2*cos(theta)^2))/100;...
	 -(cos(phi)*sin(theta)*(981*cos(theta) + 100*L*phi_dot^2 + 100*L*theta_dot^2 - 100*L*phi_dot^2*cos(theta)^2))/100;...
	 L*phi_dot^2*cos(theta)^3 - L*phi_dot^2*cos(theta) - L*theta_dot^2*cos(theta) - (981*cos(theta)^2)/100 + 981/100];
 
end
% 
function E_in = inv_E(x)
	theta		= x(5);
	phi			= x(7);
	L			= x(9); 
	
E =[1 - cos(theta)^2*sin(phi)^2 - cos(phi)^2,			cos(phi)*sin(phi) - cos(phi)*cos(theta)^2*sin(phi),	sin(phi)*sin(theta);...
	cos(phi)*sin(phi) - cos(phi)*cos(theta)^2*sin(phi),	1 - cos(phi)^2*cos(theta)^2 - sin(phi)^2,			cos(phi)*sin(theta);...
	cos(theta)*sin(phi)*sin(theta),						cos(phi)*cos(theta)*sin(theta),						cos(theta)];

E_in = inv(E);



E_BIS = [	1 - cos(theta)^2*sin(phi)^2 - cos(phi)^2,			  cos(phi)*sin(phi) - cos(phi)*cos(theta)^2*sin(phi),    sin(phi)*sin(theta);...
			cos(phi)*sin(phi) - cos(phi)*cos(theta)^2*sin(phi),				1 - cos(phi)^2*cos(theta)^2 - sin(phi)^2,    cos(phi)*sin(theta);...
            -(cos(theta)*sin(phi))/L,														-(cos(phi)*cos(theta))/L,                     0];


if rcond(E_BIS) < 1e-3
	ciao = 1;
	%rcond(E_BIS)
	%rcond(E)
end

end

== matlab function gru_FL/Generazione riferimenti/Punto/Legge Oraria ==
  data: t input; s output; v_rif parameter; dot_s output; ddot_s output
function [s, dot_s, ddot_s]  = legge_oraria(t, v_rif)
%#codegen PEPO

s = v_rif*t;
dot_s = v_rif;
ddot_s = 0.0;


end

== matlab function gru_FL/gru/x2theta_ddot ==
  data: x input; theta_ddot output; x_t_ddot input; y_t_ddot input; g parameter
function theta_ddot = fcn(x, x_t_ddot, y_t_ddot, g)
	
	theta		= x(5);
	theta_dot	= x(6);
	phi			= x(7);
	phi_dot		= x(8);
	L			= x(9);
	L_dot		= x(10);
	
theta_ddot = -2*(L_dot/L)*theta_dot+0.5*phi_dot^2*sin(2*theta)-(g/L)*sin(theta) + (-cos(theta)*sin(phi)/L)*x_t_ddot + (-cos(theta)*cos(phi)/L)*y_t_ddot;

== matlab function gru_FL/stop_sim/MATLAB Function1 ==
  data: flag output; err input; n output; n_old input; threshold parameter
function [flag, n] = stop_function(err, n_old, threshold)
	flag = 0;
	n = n_old;
	if norm(err, 2) < threshold
		n=n+1;
	else
		n=0;
	end
	
	if n > 500
		flag = 1;
		n = 0;
	end
end

== matlab function gru_FL/Generazione riferimenti/Punto/Percorso ==
  data: s input; rif output; x_M_finale parameter; x_M_iniziale parameter; y_M_finale parameter; y_M_iniziale parameter
function rif  = punto2punto(s, x_M_finale, x_M_iniziale, y_M_finale, y_M_iniziale)

vett = [x_M_finale - x_M_iniziale; y_M_finale - y_M_iniziale];
Ltot = norm(vett,2);
direzione = vett/Ltot;
offset = 0;

if s >= Ltot
	rif = [x_M_finale + offset; y_M_finale + offset];
else
	rif = [ x_M_iniziale + offset; y_M_iniziale + offset] + s * direzione;
end
% 
% if s > 2*Ltot
% 	s = mod(s, 2*Ltot);
% end
% 
% if s >= Ltot
% 	rif = [ x_M_finale ; y_M_finale ] - (s-Ltot) * direzione;
% 	
% else
% 	rif = [ x_M_iniziale ; y_M_iniziale ] + s * direzione;
% end



end
